simulink model "SecRwLtStMovConfigConvert"  (R2018b)
settings: Solver=FixedStepDiscrete  StartTime=0.0  StopTime=10.0  FixedStep=0.01  RelTol=1e-3
undefined symbols (not defined in the file or in its folder): IfKeSMSbSeatMovBkRclnEnable_Val, IfKeSMSbSeatMovFrwdBkwdEnable_Val, IfKeSMSbSeatMovFtrstEnable_Val, IfKeSMSbSeatMovHdrstFrwdBkwdEnable_Val, IfKeSMSbSeatMovHdUpwdDnwdEnable_Val, IfKeSMSbSeatMovLgrstEnable_Val, IfKeSMSbSeatMovLtwdRtwdEnable_Val, KeSMSbArmscreenMovEnable_Val, KeSMSbSeatMovLgrstExpdEnable_Val
settings Model: Creator=sn2xws  LastModifiedBy=sn2xws
settings DataIOCC: SaveFormat=StructureWithTime
settings OptimizationCC: DefaultParameterBehavior=Inlined  EnhancedBackFolding=on  PassReuseOutputArgsAs=Individual arguments  ZeroExternalMemoryAtStartup=off  ZeroInternalMemoryAtStartup=off  OptimizeBlockOrder=speed  DifferentSizesBufferReuse=on  OptimizationCustomize=off
settings DebuggingCC: ParameterTunabilityLossMsg=error
settings ModelReferenceCC: ModelReferenceNumInstancesAllowed=Single
settings SFSimCC: MATLABDynamicMemAlloc=off
settings RTWCC: SystemTargetFile=autosar.tlc  GenCodeOnly=on  TemplateMakefile=ert_default_tmf  Description=AUTOSAR  GenerateReport=on  IncludeHyperlinkInReport=on  LaunchReport=on  GenerateTraceInfo=on  GenerateTraceReport=on  GenerateTraceReportSl=on  GenerateTraceReportSf=on  GenerateTraceReportEml=on
settings CodeAppCC: ForceParamTrailComments=on  IgnoreCustomStorageClasses=off  OperatorAnnotations=on  SimulinkDataObjDesc=on  SFDataObjDesc=on  InsertBlockDesc=on
settings STFCustomTargetCC: TargetLangStandard=C99 (ISO)  MultiwordLength=256  ParMdlRefBuildCompliant=on  CompOptLevelCompliant=on  IncludeMdlTerminateFcn=off  CombineOutputUpdateFcns=on  SuppressErrorStatus=on  ERTCustomFileBanners=on  SupportNonFinite=off  SupportComplex=off  SupportContinuousTime=off  SupportNonInlinedSFcns=off  RemoveResetFunc=on  MATLABClassNameForMDSCustomization=Simulink.SoftwareTarget.ERTCustomization  AutosarCompliant=on  UseToolchainInfoCompliant=on  LookupTableObjectStructAxisOrder=2,1,3,4,...  LUTObjectStructOrderEvenSpacing=Size,Table,Breakpoints  SystemTargetFile=autosar.tlc
settings ERTTargetCC: TargetLangStandard=C99 (ISO)  ConcurrentExecutionCompliant=off  IncludeMdlTerminateFcn=off  SuppressErrorStatus=on  SupportNonFinite=off  SupportComplex=off  ModelStepFunctionPrototypeControlCompliant=off  CPPClassGenCompliant=off  AutosarCompliant=on  LookupTableObjectStructAxisOrder=2,1,3,4,...  LUTObjectStructOrderEvenSpacing=Size,Table,Breakpoints  InlinedParameterPlacement=NonHierarchical  ERTCustomFileTemplate=example_file_process.tlc  ERTFilePackagingFormat=Compact

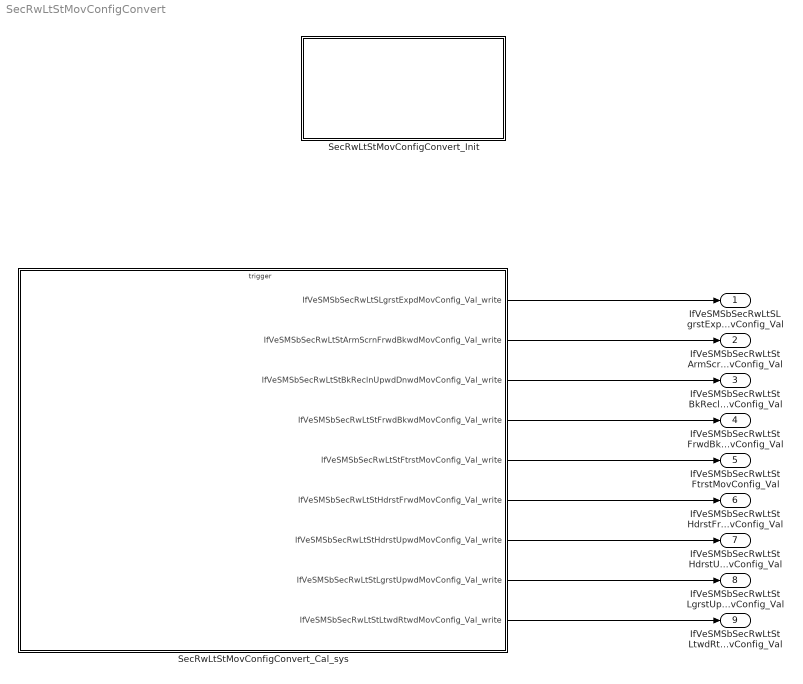
== system SecRwLtStMovConfigConvert ==
  SecRwLtStMovConfigConvert_Cal_sys : Subsystem
  SecRwLtStMovConfigConvert_Init : Subsystem
  IfVeSMSbSecRwLtSLgrstExpdMovConfig_Val : Outport  OutDataTypeStr=boolean  PortDimensions=1
  IfVeSMSbSecRwLtStArmScrnFrwdBkwdMovConfig_Val : Outport  Port=2  OutDataTypeStr=boolean  PortDimensions=1
  IfVeSMSbSecRwLtStBkReclnUpwdDnwdMovConfig_Val : Outport  Port=3  OutDataTypeStr=boolean  PortDimensions=1
  IfVeSMSbSecRwLtStFrwdBkwdMovConfig_Val : Outport  Port=4  OutDataTypeStr=boolean  PortDimensions=1
  IfVeSMSbSecRwLtStFtrstMovConfig_Val : Outport  Port=5  OutDataTypeStr=boolean  PortDimensions=1
  IfVeSMSbSecRwLtStHdrstFrwdMovConfig_Val : Outport  Port=6  OutDataTypeStr=boolean  PortDimensions=1
  IfVeSMSbSecRwLtStHdrstUpwdMovConfig_Val : Outport  Port=7  OutDataTypeStr=boolean  PortDimensions=1
  IfVeSMSbSecRwLtStLgrstUpwdMovConfig_Val : Outport  Port=8  OutDataTypeStr=boolean  PortDimensions=1
  IfVeSMSbSecRwLtStLtwdRtwdMovConfig_Val : Outport  Port=9  OutDataTypeStr=boolean  PortDimensions=1
  wires:
  SecRwLtStMovConfigConvert_Cal_sys/1(IfVeSMSbSecRwLtSLgrstExpdMovConfig_Val_write) -> IfVeSMSbSecRwLtSLgrstExpdMovConfig_Val/1
  SecRwLtStMovConfigConvert_Cal_sys/2(IfVeSMSbSecRwLtStArmScrnFrwdBkwdMovConfig_Val_write) -> IfVeSMSbSecRwLtStArmScrnFrwdBkwdMovConfig_Val/1
  SecRwLtStMovConfigConvert_Cal_sys/3(IfVeSMSbSecRwLtStBkReclnUpwdDnwdMovConfig_Val_write) -> IfVeSMSbSecRwLtStBkReclnUpwdDnwdMovConfig_Val/1
  SecRwLtStMovConfigConvert_Cal_sys/4(IfVeSMSbSecRwLtStFrwdBkwdMovConfig_Val_write) -> IfVeSMSbSecRwLtStFrwdBkwdMovConfig_Val/1
  SecRwLtStMovConfigConvert_Cal_sys/5(IfVeSMSbSecRwLtStFtrstMovConfig_Val_write) -> IfVeSMSbSecRwLtStFtrstMovConfig_Val/1
  SecRwLtStMovConfigConvert_Cal_sys/6(IfVeSMSbSecRwLtStHdrstFrwdMovConfig_Val_write) -> IfVeSMSbSecRwLtStHdrstFrwdMovConfig_Val/1
  SecRwLtStMovConfigConvert_Cal_sys/7(IfVeSMSbSecRwLtStHdrstUpwdMovConfig_Val_write) -> IfVeSMSbSecRwLtStHdrstUpwdMovConfig_Val/1
  SecRwLtStMovConfigConvert_Cal_sys/8(IfVeSMSbSecRwLtStLgrstUpwdMovConfig_Val_write) -> IfVeSMSbSecRwLtStLgrstUpwdMovConfig_Val/1
  SecRwLtStMovConfigConvert_Cal_sys/9(IfVeSMSbSecRwLtStLtwdRtwdMovConfig_Val_write) -> IfVeSMSbSecRwLtStLtwdRtwdMovConfig_Val/1

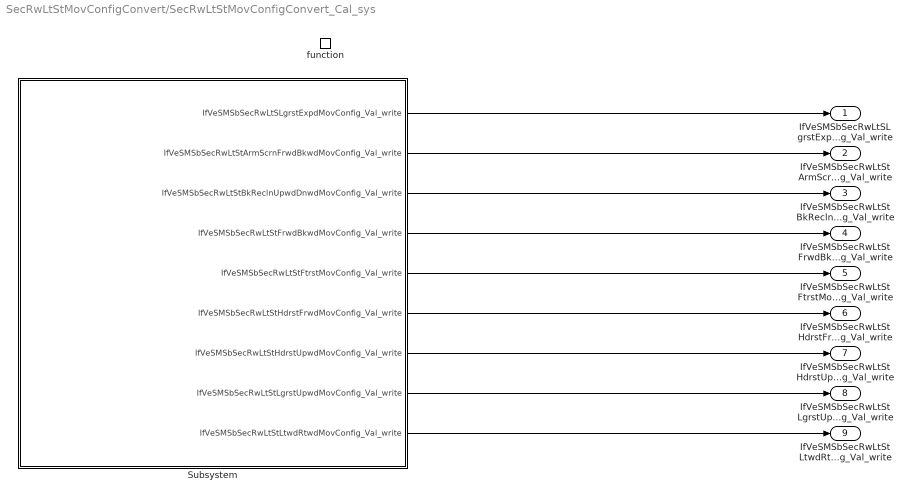
== system SecRwLtStMovConfigConvert/SecRwLtStMovConfigConvert_Cal_sys ==
  function : TriggerPort  TriggerType=function-call  IsSimulinkFunction=on  FunctionName=SecRwLtStMovConfigConvert_Cal  VariantControl=(inherit)
  Subsystem : Subsystem
  IfVeSMSbSecRwLtSLgrstExpdMovConfig_Val_write : Outport
      settings: EnsureOutportIsVirtual=on
  IfVeSMSbSecRwLtStArmScrnFrwdBkwdMovConfig_Val_write : Outport  Port=2
      settings: EnsureOutportIsVirtual=on
  IfVeSMSbSecRwLtStBkReclnUpwdDnwdMovConfig_Val_write : Outport  Port=3
      settings: EnsureOutportIsVirtual=on
  IfVeSMSbSecRwLtStFrwdBkwdMovConfig_Val_write : Outport  Port=4
      settings: EnsureOutportIsVirtual=on
  IfVeSMSbSecRwLtStFtrstMovConfig_Val_write : Outport  Port=5
      settings: EnsureOutportIsVirtual=on
  IfVeSMSbSecRwLtStHdrstFrwdMovConfig_Val_write : Outport  Port=6
      settings: EnsureOutportIsVirtual=on
  IfVeSMSbSecRwLtStHdrstUpwdMovConfig_Val_write : Outport  Port=7
      settings: EnsureOutportIsVirtual=on
  IfVeSMSbSecRwLtStLgrstUpwdMovConfig_Val_write : Outport  Port=8
      settings: EnsureOutportIsVirtual=on
  IfVeSMSbSecRwLtStLtwdRtwdMovConfig_Val_write : Outport  Port=9
      settings: EnsureOutportIsVirtual=on
  wires:
  Subsystem/6(IfVeSMSbSecRwLtStHdrstFrwdMovConfig_Val_write) -> IfVeSMSbSecRwLtStHdrstFrwdMovConfig_Val_write/1
  Subsystem/7(IfVeSMSbSecRwLtStHdrstUpwdMovConfig_Val_write) -> IfVeSMSbSecRwLtStHdrstUpwdMovConfig_Val_write/1
  Subsystem/8(IfVeSMSbSecRwLtStLgrstUpwdMovConfig_Val_write) -> IfVeSMSbSecRwLtStLgrstUpwdMovConfig_Val_write/1
  Subsystem/4(IfVeSMSbSecRwLtStFrwdBkwdMovConfig_Val_write) -> IfVeSMSbSecRwLtStFrwdBkwdMovConfig_Val_write/1
  Subsystem/5(IfVeSMSbSecRwLtStFtrstMovConfig_Val_write) -> IfVeSMSbSecRwLtStFtrstMovConfig_Val_write/1
  Subsystem/9(IfVeSMSbSecRwLtStLtwdRtwdMovConfig_Val_write) -> IfVeSMSbSecRwLtStLtwdRtwdMovConfig_Val_write/1
  Subsystem/1(IfVeSMSbSecRwLtSLgrstExpdMovConfig_Val_write) -> IfVeSMSbSecRwLtSLgrstExpdMovConfig_Val_write/1
  Subsystem/2(IfVeSMSbSecRwLtStArmScrnFrwdBkwdMovConfig_Val_write) -> IfVeSMSbSecRwLtStArmScrnFrwdBkwdMovConfig_Val_write/1
  Subsystem/3(IfVeSMSbSecRwLtStBkReclnUpwdDnwdMovConfig_Val_write) -> IfVeSMSbSecRwLtStBkReclnUpwdDnwdMovConfig_Val_write/1

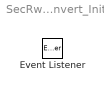
== system SecRwLtStMovConfigConvert/SecRwLtStMovConfigConvert_Init ==
  Event Listener : EventListener  EventName=reset

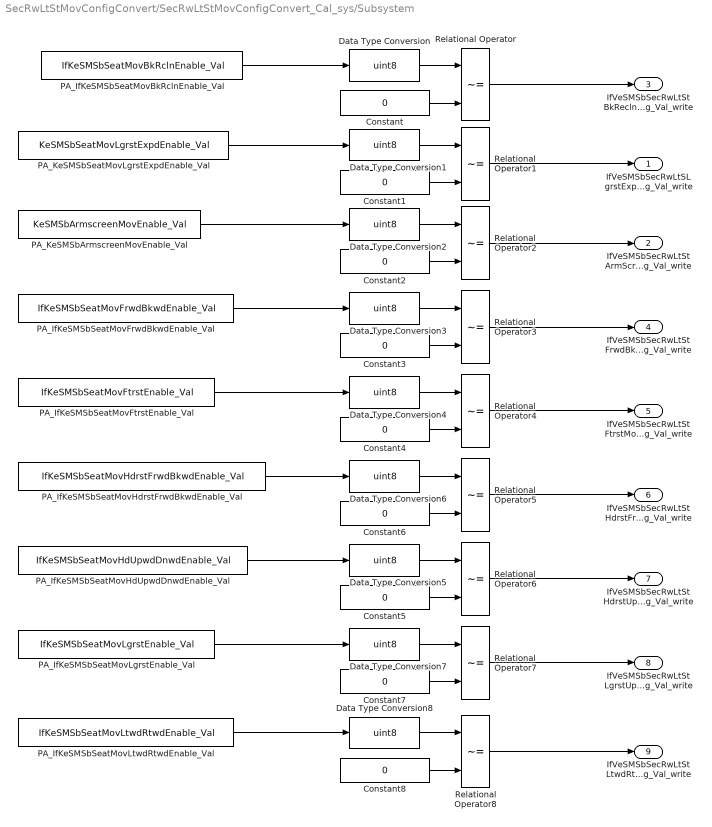
== system SecRwLtStMovConfigConvert/SecRwLtStMovConfigConvert_Cal_sys/Subsystem ==
  Constant{,1..8} (9 alike) : Constant  Value=0
  Data Type Conversion{,1..8} (9 alike) : DataTypeConversion  OutDataTypeStr=uint8
  PA_IfKeSMSbSeatMovBkRclnEnable_Val : Constant  Value=IfKeSMSbSeatMovBkRclnEnable_Val
  PA_IfKeSMSbSeatMovFrwdBkwdEnable_Val : Constant  Value=IfKeSMSbSeatMovFrwdBkwdEnable_Val
  PA_IfKeSMSbSeatMovFtrstEnable_Val : Constant  Value=IfKeSMSbSeatMovFtrstEnable_Val
  PA_IfKeSMSbSeatMovHdUpwdDnwdEnable_Val : Constant  Value=IfKeSMSbSeatMovHdUpwdDnwdEnable_Val
  PA_IfKeSMSbSeatMovHdrstFrwdBkwdEnable_Val : Constant  Value=IfKeSMSbSeatMovHdrstFrwdBkwdEnable_Val
  PA_IfKeSMSbSeatMovLgrstEnable_Val : Constant  Value=IfKeSMSbSeatMovLgrstEnable_Val
  PA_IfKeSMSbSeatMovLtwdRtwdEnable_Val : Constant  Value=IfKeSMSbSeatMovLtwdRtwdEnable_Val
  PA_KeSMSbArmscreenMovEnable_Val : Constant  Value=KeSMSbArmscreenMovEnable_Val
  PA_KeSMSbSeatMovLgrstExpdEnable_Val : Constant  Value=KeSMSbSeatMovLgrstExpdEnable_Val
  Relational Operator{,1..8} (9 alike) : RelationalOperator  Operator=~=  OutDataTypeStr=boolean  RndMeth=Simplest
  IfVeSMSbSecRwLtSLgrstExpdMovConfig_Val_write : Outport
      settings: EnsureOutportIsVirtual=on
  IfVeSMSbSecRwLtStArmScrnFrwdBkwdMovConfig_Val_write : Outport  Port=2
      settings: EnsureOutportIsVirtual=on
  IfVeSMSbSecRwLtStBkReclnUpwdDnwdMovConfig_Val_write : Outport  Port=3
      settings: EnsureOutportIsVirtual=on
  IfVeSMSbSecRwLtStFrwdBkwdMovConfig_Val_write : Outport  Port=4
      settings: EnsureOutportIsVirtual=on
  IfVeSMSbSecRwLtStFtrstMovConfig_Val_write : Outport  Port=5
      settings: EnsureOutportIsVirtual=on
  IfVeSMSbSecRwLtStHdrstFrwdMovConfig_Val_write : Outport  Port=6
      settings: EnsureOutportIsVirtual=on
  IfVeSMSbSecRwLtStHdrstUpwdMovConfig_Val_write : Outport  Port=7
      settings: EnsureOutportIsVirtual=on
  IfVeSMSbSecRwLtStLgrstUpwdMovConfig_Val_write : Outport  Port=8
      settings: EnsureOutportIsVirtual=on
  IfVeSMSbSecRwLtStLtwdRtwdMovConfig_Val_write : Outport  Port=9
      settings: EnsureOutportIsVirtual=on
  wires:
  PA_IfKeSMSbSeatMovBkRclnEnable_Val/1 -> Data Type Conversion/1
  Constant/1 -> Relational Operator/2
  Data Type Conversion/1 -> Relational Operator/1
  Relational Operator/1 -> IfVeSMSbSecRwLtStBkReclnUpwdDnwdMovConfig_Val_write/1
  Data Type Conversion1/1 -> Relational Operator1/1
  Constant1/1 -> Relational Operator1/2
  PA_KeSMSbSeatMovLgrstExpdEnable_Val/1 -> Data Type Conversion1/1
  Relational Operator1/1 -> IfVeSMSbSecRwLtSLgrstExpdMovConfig_Val_write/1
  Relational Operator2/1 -> IfVeSMSbSecRwLtStArmScrnFrwdBkwdMovConfig_Val_write/1
  PA_KeSMSbArmscreenMovEnable_Val/1 -> Data Type Conversion2/1
  Constant2/1 -> Relational Operator2/2
  Data Type Conversion2/1 -> Relational Operator2/1
  Data Type Conversion3/1 -> Relational Operator3/1
  Constant3/1 -> Relational Operator3/2
  PA_IfKeSMSbSeatMovFrwdBkwdEnable_Val/1 -> Data Type Conversion3/1
  PA_IfKeSMSbSeatMovFtrstEnable_Val/1 -> Data Type Conversion4/1
  Constant4/1 -> Relational Operator4/2
  Data Type Conversion4/1 -> Relational Operator4/1
  Data Type Conversion5/1 -> Relational Operator6/1
  Constant5/1 -> Relational Operator6/2
  PA_IfKeSMSbSeatMovHdUpwdDnwdEnable_Val/1 -> Data Type Conversion5/1
  PA_IfKeSMSbSeatMovHdrstFrwdBkwdEnable_Val/1 -> Data Type Conversion6/1
  Data Type Conversion6/1 -> Relational Operator5/1
  Constant6/1 -> Relational Operator5/2
  PA_IfKeSMSbSeatMovLgrstEnable_Val/1 -> Data Type Conversion7/1
  Constant7/1 -> Relational Operator7/2
  Data Type Conversion7/1 -> Relational Operator7/1
  Data Type Conversion8/1 -> Relational Operator8/1
  Constant8/1 -> Relational Operator8/2
  PA_IfKeSMSbSeatMovLtwdRtwdEnable_Val/1 -> Data Type Conversion8/1
  Relational Operator3/1 -> IfVeSMSbSecRwLtStFrwdBkwdMovConfig_Val_write/1
  Relational Operator4/1 -> IfVeSMSbSecRwLtStFtrstMovConfig_Val_write/1
  Relational Operator5/1 -> IfVeSMSbSecRwLtStHdrstFrwdMovConfig_Val_write/1
  Relational Operator6/1 -> IfVeSMSbSecRwLtStHdrstUpwdMovConfig_Val_write/1
  Relational Operator7/1 -> IfVeSMSbSecRwLtStLgrstUpwdMovConfig_Val_write/1
  Relational Operator8/1 -> IfVeSMSbSecRwLtStLtwdRtwdMovConfig_Val_write/1
